simulink model "RealModelWithFlexLoadX1X2X3"  (R2019a)
settings: Solver=ode4  StartTime=0.0  StopTime=50  FixedStep=1e-4  MaxStep=1e-4  MinStep=1e-6  RelTol=1e-10
InitFcn:
  | Rs = 0.011
  | Ld = 0.018
  | Lq = 0.018
  | Fi = 0.055
  | p = 4
  | J = 0.102
  | b = 0.18
  | 
  | A1 = 1
  | B1 = -5000
  | B2 = -0.0200
  | B3 = 10
  | C1 = 500
  | C2 = -2.499999800000000e+04
  | C3 = -90.999999999999990
  | C4 = 110
  | 
  | tC = 50
  | k3 = -1.620402364619914
  | k4 = -0.507865883970218
  | k5 = -0.507865883970218
  | k6 = -0.294132929497733
  | 
  | ide = 3.024305555555556
  | iqe = 0.307424053403619
  | 
  | tO = 20
  | g1 = 0.164052784000000
  | g2 = -2.996000000000000
  | g3 = 8.089800000000000e+02
settings Model: Creator=LiLid  LastModifiedBy=LiLid

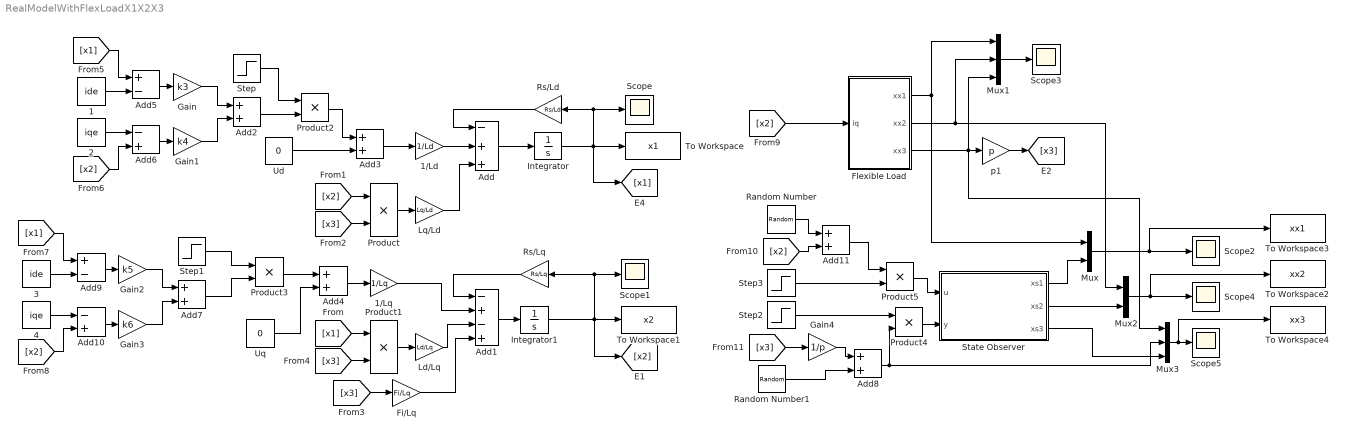
== system RealModelWithFlexLoadX1X2X3 ==
  1 : Constant  Value=ide
  1/Ld : Gain  Gain=1/Ld
  1/Lq : Gain  Gain=1/Lq
  2 : Constant  Value=iqe
  3 : Constant  Value=ide
  4 : Constant  Value=iqe
  Add : Sum  Inputs=-++
  Add1 : Sum  Inputs=-+-+
  Add10 : Sum  Inputs=-+
  Add{2..4,7..8,11} (6 alike) : Sum
  Add5 : Sum  Inputs=+-
  Add6 : Sum  Inputs=-+
  Add9 : Sum  Inputs=+-
  Fi/Lq : Gain  Gain=Fi/Lq
  Flexible Load : Subsystem
  Gain : Gain  Gain=k3
  Gain1 : Gain  Gain=k4
  Gain2 : Gain  Gain=k5
  Gain3 : Gain  Gain=k6
  Gain4 : Gain  Gain=1/p
  Integrator : Integrator  InitialCondition=1
  Integrator1 : Integrator  InitialCondition=1
  Ld/Lq : Gain  Gain=Ld/Lq
  Lq/Ld : Gain  Gain=Lq/Ld
  Mux : Mux  Inputs=2
  Mux1 : Mux  Inputs=3
  Mux2 : Mux  Inputs=2
  Mux3 : Mux  Inputs=3
  Product{,1..5} (6 alike) : Product
  Random Number : RandomNumber  Variance=0.1  SampleTime=0.0001
  Random Number1 : RandomNumber  Variance=0.1  SampleTime=0.0001
  Rs/Ld : Gain  Gain=Rs/Ld
  Rs/Lq : Gain  Gain=Rs/Lq
  Scope{,1..5} (6 alike) : Scope
  State Observer : Subsystem
  Step : Step  Time=tC  SampleTime=0
  Step1 : Step  Time=tC  SampleTime=0
  Step2 : Step  Time=tO  SampleTime=0
  Step3 : Step  Time=tO  SampleTime=0
  To Workspace : ToWorkspace  VariableName=x1  SampleTime=-1
      settings: Save2DSignal=2-D array (concatenate along first dimension)
  To Workspace1 : ToWorkspace  VariableName=x2  SampleTime=-1
      settings: Save2DSignal=2-D array (concatenate along first dimension)
  To Workspace2 : ToWorkspace  VariableName=xx2  SampleTime=-1
      settings: Save2DSignal=2-D array (concatenate along first dimension)
  To Workspace3 : ToWorkspace  VariableName=xx1  SampleTime=-1
      settings: Save2DSignal=2-D array (concatenate along first dimension)
  To Workspace4 : ToWorkspace  VariableName=xx3  SampleTime=-1
      settings: Save2DSignal=2-D array (concatenate along first dimension)
  Ud : Constant  Value=0
  Uq : Constant  Value=0
  p1 : Gain  Gain=p
  wires:
  Integrator/1 -> To Workspace/1, [x1], Scope/1, Rs/Ld/1
  Add/1 -> Integrator/1
  Rs/Ld/1 -> Add/1
  Product/1 -> Lq/Ld/1
  [x2] -> Product/1
  [x3] -> Product/2
  Integrator1/1 -> To Workspace1/1, Rs/Lq/1, Scope1/1, [x2]
  Rs/Lq/1 -> Add1/1
  Add1/1 -> Integrator1/1
  [x1] -> Product1/1
  [x3] -> Product1/2
  [x3] -> Fi/Lq/1
  Fi/Lq/1 -> Add1/4
  Lq/Ld/1 -> Add/3
  1/Ld/1 -> Add/2
  1/Lq/1 -> Add1/2
  Product1/1 -> Ld/Lq/1
  Ld/Lq/1 -> Add1/3
  Gain1/1 -> Add2/2
  Gain/1 -> Add2/1
  Add2/1 -> Product2/2
  Ud/1 -> Add3/2
  Add3/1 -> 1/Ld/1
  Step/1 -> Product2/1
  Product2/1 -> Add3/1
  Add4/1 -> 1/Lq/1
  Uq/1 -> Add4/2
  Product3/1 -> Add4/1
  Add5/1 -> Gain/1
  [x1] -> Add5/1
  1/1 -> Add5/2
  Add6/1 -> Gain1/1
  2/1 -> Add6/1
  [x2] -> Add6/2
  3/1 -> Add9/2
  [x2] -> Add10/2
  4/1 -> Add10/1
  Gain2/1 -> Add7/1
  Add10/1 -> Gain3/1
  [x1] -> Add9/1
  Add9/1 -> Gain2/1
  Gain3/1 -> Add7/2
  Add7/1 -> Product3/2
  Step1/1 -> Product3/1
  [x2] -> Flexible Load/1(iq)
  Flexible Load/3(xx3) -> Mux3/1, Mux1/3, p1/1
  p1/1 -> [x3]
  [x3] -> Gain4/1
  Step2/1 -> Product4/1
  Step3/1 -> Product5/2
  Mux/1 -> To Workspace3/1, Scope2/1
  Product5/1 -> State Observer/1(u)
  Product4/1 -> State Observer/2(y)
  Flexible Load/2(xx2) -> Mux1/2, Mux2/1
  Flexible Load/1(xx1) -> Mux1/1, Mux/1
  Mux1/1 -> Scope3/1
  State Observer/1(xs1) -> Mux/2
  State Observer/2(xs2) -> Mux2/2
  Mux2/1 -> To Workspace2/1, Scope4/1
  Mux3/1 -> To Workspace4/1, Scope5/1
  Random Number1/1 -> Add8/2
  Random Number/1 -> Add11/1
  [x2] -> Add11/2
  Add11/1 -> Product5/1
  Gain4/1 -> Add8/1
  Add8/1 -> Product4/2, Mux3/2
  State Observer/3(xs3) -> Mux3/3

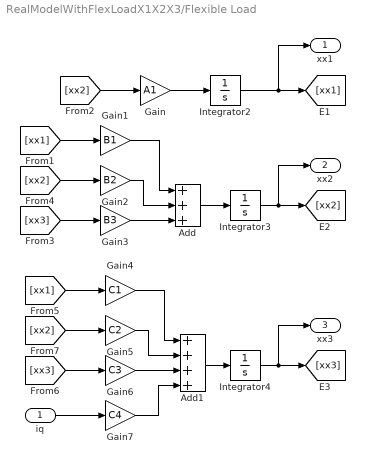
== system RealModelWithFlexLoadX1X2X3/Flexible Load ==
  iq : Inport
  Add : Sum  Inputs=+++
  Add1 : Sum  Inputs=++++
  Gain : Gain  Gain=A1
  Gain1 : Gain  Gain=B1
  Gain2 : Gain  Gain=B2
  Gain3 : Gain  Gain=B3
  Gain4 : Gain  Gain=C1
  Gain5 : Gain  Gain=C2
  Gain6 : Gain  Gain=C3
  Gain7 : Gain  Gain=C4
  Integrator2 : Integrator
  Integrator3 : Integrator
  Integrator4 : Integrator
  xx1 : Outport
  xx2 : Outport  Port=2
  xx3 : Outport  Port=3
  wires:
  Integrator2/1 -> xx1/1, [xx1]
  Integrator3/1 -> [xx2], xx2/1
  Integrator4/1 -> xx3/1, [xx3]
  [xx2] -> Gain/1
  Gain/1 -> Integrator2/1
  [xx1] -> Gain1/1
  [xx2] -> Gain2/1
  [xx3] -> Gain3/1
  Add/1 -> Integrator3/1
  Gain3/1 -> Add/3
  Gain2/1 -> Add/2
  Gain1/1 -> Add/1
  [xx1] -> Gain4/1
  [xx2] -> Gain5/1
  Add1/1 -> Integrator4/1
  Gain5/1 -> Add1/2
  [xx3] -> Gain6/1
  Gain6/1 -> Add1/3
  Gain4/1 -> Add1/1
  iq/1 -> Gain7/1
  Gain7/1 -> Add1/4

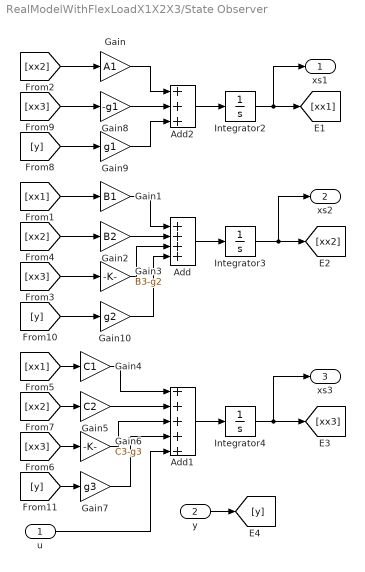
== system RealModelWithFlexLoadX1X2X3/State Observer ==
  u : Inport
  y : Inport  Port=2
  Add : Sum  Inputs=++++
  Add1 : Sum  Inputs=+++++
  Add2 : Sum  Inputs=+++
  Gain : Gain  Gain=A1
  Gain1 : Gain  Gain=B1
  Gain10 : Gain  Gain=g2
  Gain2 : Gain  Gain=B2
  Gain3 : Gain  Gain=B3-g2
  Gain4 : Gain  Gain=C1
  Gain5 : Gain  Gain=C2
  Gain6 : Gain  Gain=C3-g3
  Gain7 : Gain  Gain=g3
  Gain8 : Gain  Gain=-g1
  Gain9 : Gain  Gain=g1
  Integrator2 : Integrator
  Integrator3 : Integrator
  Integrator4 : Integrator
  xs1 : Outport
  xs2 : Outport  Port=2
  xs3 : Outport  Port=3
  wires:
  Integrator3/1 -> [xx2], xs2/1
  Integrator4/1 -> [xx3], xs3/1
  [xx2] -> Gain/1
  [xx1] -> Gain1/1
  [xx2] -> Gain2/1
  [xx3] -> Gain3/1
  Add/1 -> Integrator3/1
  Gain3/1 -> Add/3
  Gain2/1 -> Add/2
  Gain1/1 -> Add/1
  [xx1] -> Gain4/1
  [xx2] -> Gain5/1
  Add1/1 -> Integrator4/1
  Gain5/1 -> Add1/2
  [xx3] -> Gain6/1
  Gain6/1 -> Add1/3
  Gain4/1 -> Add1/1
  Gain7/1 -> Add1/4
  y/1 -> [y]
  [xx3] -> Gain8/1
  [y] -> Gain9/1
  Gain8/1 -> Add2/2
  Gain9/1 -> Add2/3
  Gain/1 -> Add2/1
  Add2/1 -> Integrator2/1
  Integrator2/1 -> xs1/1, [xx1]
  Gain10/1 -> Add/4
  [y] -> Gain10/1
  [y] -> Gain7/1
  u/1 -> Add1/5
